simulink model "linear_model"  (R2020b)
settings: Solver=VariableStepAuto  StartTime=0  StopTime=2  RelTol=1e-3
values from neighbouring files (symbols this model uses):
  alphar = poly2sym(y3,t)    [lpv_model.m]
  hr = poly2sym(y6,t)    [lpv_model.m]
  miur = poly2sym(y2,t)    [lpv_model.m]
  qr = poly2sym(y4,t)    [lpv_model.m]
  Vr = poly2sym(y1,t)    [lpv_model.m]
  xr = poly2sym(y5,t)    [lpv_model.m]    (also in xr(0.0.01.2).mat = [9.97354758391 9.97900733809 9.98348279699 9.98718538751 9.9)
settings Model: Creator=Lenovo  LastModifiedBy=Eric
settings DataIOCC: ReturnWorkspaceOutputs=off
settings OptimizationCC: LifeSpan=inf
settings DebuggingCC: ArithmeticOperatorsInVariantConditions=warning
settings SFSimCC: CustomCodeUndefinedFunction=UseInterfaceOnly
settings CodeAppCC: StateflowObjectComments=on

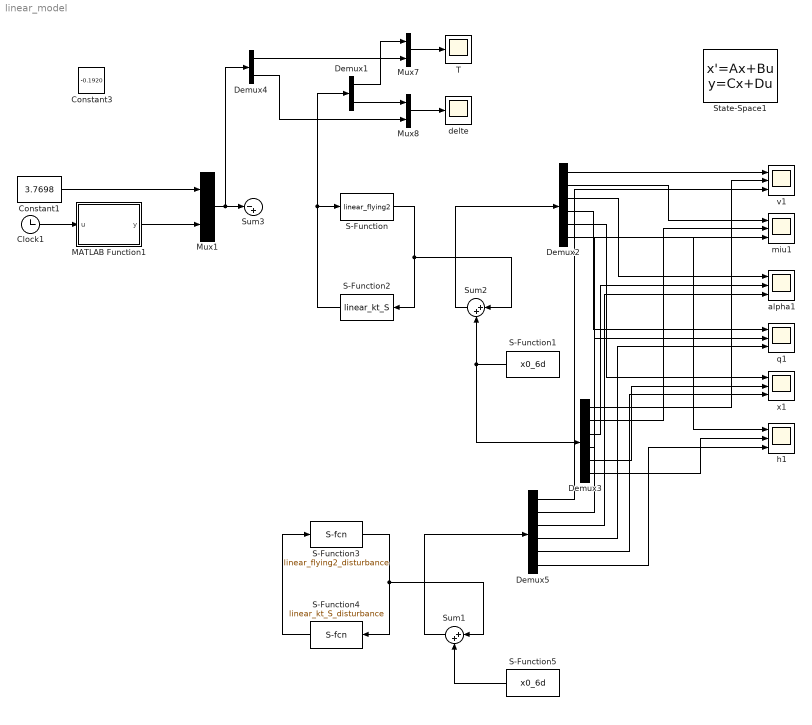
== system linear_model ==
  Clock1 : Clock
  Constant1 : Constant  Value=3.7698
  Constant3 : Constant  Value=-0.1920
  Demux1 : Demux  Outputs=2
  Demux2 : Demux  Outputs=6
  Demux3 : Demux  Outputs=6
  Demux4 : Demux  Outputs=2
  Demux5 : Demux  Outputs=6
  MATLAB Function1 : MATLAB Function  TreatAsAtomicUnit=on
  Mux1 : Mux  Inputs=2
  Mux7 : Mux  Inputs=2
  Mux8 : Mux  Inputs=2
  S-Function : S-Function  FunctionName=linear_flying2  Parameters=A_all, B_all  SFunctionDeploymentMode=off  EnableBusSupport=off
  S-Function1 : S-Function  FunctionName=x0_6d  Parameters=Vr,miur,alphar,qr,xr,hr  SFunctionDeploymentMode=off  EnableBusSupport=off
  S-Function2 : S-Function  FunctionName=linear_kt_S  Parameters=Kall  SFunctionDeploymentMode=off  EnableBusSupport=off
  S-Function3 : S-Function  FunctionName=linear_flying2_disturbance  Parameters=A_all1, B_all1  SFunctionDeploymentMode=off  EnableBusSupport=off
  S-Function4 : S-Function  FunctionName=linear_kt_S_disturbance  Parameters=Kall1  SFunctionDeploymentMode=off  EnableBusSupport=off
  S-Function5 : S-Function  FunctionName=x0_6d  Parameters=Vr,miur,alphar,qr,xr,hr  SFunctionDeploymentMode=off  EnableBusSupport=off
  State-Space1 : StateSpace  A="[-0.874195781546103\t-9.79991342327446\t-16.9317089290089\t0\t0\t0;0.177469289690789\t0.00413618626824430\t3.70308454827272\t0\t0\t0;-0.177469289722834\t-0.00413618752312663\t-3.70308454866770\t0.999999999999999\t0\t0;-0.190303547702634\t0\t-12.7586792403921\t0\t0\t0;0.999991178208150\t-0.0418034523312236\t0\t0\t0\t0;0.00420041728281824\t9.95211136705568\t0\t0\t0\t0]"  B="[1.20975427644587\t0;0.0316145255023421\t0;-0.0316145255023414\t0;0\t12.1661211931646;0 0;0 0]"  C=[1 0 0 0 0 0;0 1 0 0 0 0;0 0 1 0 0 0;0 0 0 1 0 0;0 0 0 0 1 0;0 0 0 0 0 1]  D=[0 0;0 0;0 0;0 0;0 0;0 0]  InitialCondition="[11  0.1  0.3  0.1  1 -1]"
  Sum1 : Sum  Inputs=|++
  Sum2 : Sum  Inputs=|++
  Sum3 : Sum  Inputs=|-+
  T : Scope
  alpha1 : Scope  NumInputPorts=3
  delte : Scope
  h1 : Scope  NumInputPorts=3
  miu1 : Scope  NumInputPorts=3
  q1 : Scope  NumInputPorts=3
  v1 : Scope  NumInputPorts=3
  x1 : Scope  NumInputPorts=3
  wires:
  Demux2/5 -> x1/1
  Demux3/4 -> q1/2
  Demux2/2 -> miu1/1
  Demux3/6 -> h1/2
  Demux3/1 -> v1/2
  Demux2/3 -> alpha1/1
  Demux2/1 -> v1/1
  Demux2/4 -> q1/1
  Demux3/2 -> miu1/2
  Demux2/6 -> h1/1
  Demux3/3 -> alpha1/2
  Demux3/5 -> x1/2
  Mux8/1 -> delte/1
  Mux7/1 -> T/1
  Clock1/1 -> MATLAB Function1/1(u)
  MATLAB Function1/1(y) -> Mux1/2
  Constant1/1 -> Mux1/1
  Demux1/2 -> Mux8/1
  Demux4/2 -> Mux8/2
  Demux4/1 -> Mux7/2
  Demux1/1 -> Mux7/1
  Mux1/1 -> Sum3/1, Demux4/1
  S-Function2/1 -> Demux1/1, S-Function/1
  S-Function1/1 -> Sum2/2, Demux3/1
  S-Function/1 -> S-Function2/1, Sum2/1
  Sum2/1 -> Demux2/1
  S-Function4/1 -> S-Function3/1
  Sum1/1 -> Demux5/1
  S-Function3/1 -> Sum1/1, S-Function4/1
  S-Function5/1 -> Sum1/2
  Demux5/1 -> v1/3
  Demux5/2 -> miu1/3
  Demux5/3 -> alpha1/3
  Demux5/4 -> q1/3
  Demux5/5 -> x1/3
  Demux5/6 -> h1/3

== matlab function linear_model/MATLAB Function1 ==
  data: u input; y output
function y = fcn(u)
if u<0.3
    y=-(11+(u)/0.3*22)/180*pi;
else if u>=0.3&&u<0.5
        y=-(33+(u-0.3)/0.2*15)/180*pi;
else if u>=0.5&&u<0.7
        y=-(33+15-(u-0.5)/0.2*30)/180*pi;   
    else
        y=-(18)/180*pi;
    end
    end
end
